simulink model "Vending_Machine"  (R2020a)
settings: Solver=VariableStepAuto  StartTime=0.0  StopTime=10.0  RelTol=1e-3
settings Model: Creator=Shivam  LastModifiedBy=Shivam

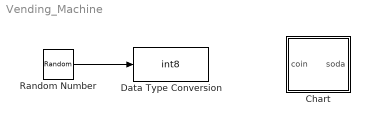
== system Vending_Machine ==
  Chart : Stateflow chart  TreatAsAtomicUnit=on
  Data Type Conversion : DataTypeConversion  OutDataTypeStr=int8
  Random Number : RandomNumber  SampleTime=0.1
  wires:
  Random Number/1 -> Data Type Conversion/1

== stateflow chart Vending_Machine/Chart ==
  state got_0
  state Got_nickel
  state Got_dime
  (default) -> got_0
  got_0 -> Got_nickel [order 1] : [coin ==1]{soda=0}
  Got_nickel -> got_0 [order 2] : [coin == 2]{soda = 1}
  Got_dime -> got_0 [order 1] : [coin ==1]{soda =1}
  got_0 -> Got_dime [order 2] : [coin == 2]{soda = 0}
  Got_nickel -> Got_dime [order 1] : [coin ==1]{soda = 0}
  Got_dime -> Got_nickel [order 2] : [coin == 2]{soda =1}
  data: coin input; soda output
